simulink model "smc_diff_with_plant_new"  (R2024b)
settings: Solver=ode1  StartTime=0.0  StopTime=30  FixedStep=1e-5  RelTol=1e-3
libraries: simulink x1
settings Model: Creator=user  LastModifiedBy=user

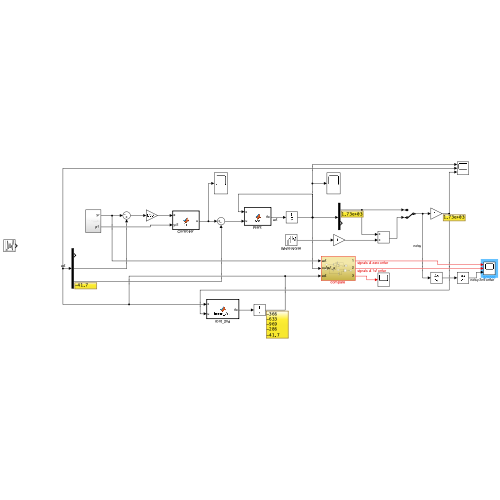
[thumbnail: Simulink's stored preview of the top-level diagram]
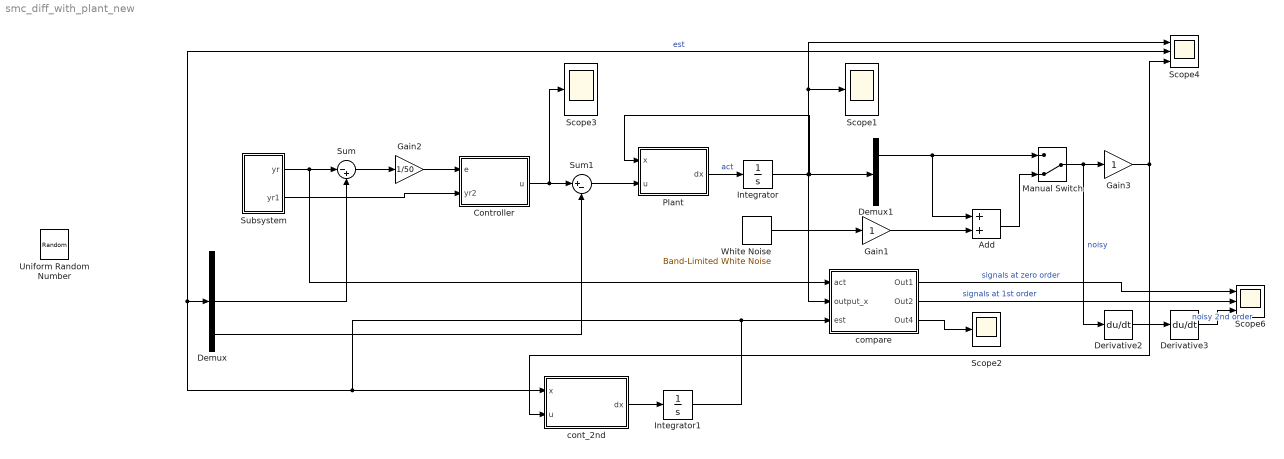
== system smc_diff_with_plant_new ==
  Add : Sum
  Controller : MATLAB Function  TreatAsAtomicUnit=on
  Demux : Demux  Outputs=[2, 2, 1]
  Demux1 : Demux  Outputs=[1, 2]
  Derivative2 : Derivative
  Derivative3 : Derivative
  Gain1 : Gain
  Gain2 : Gain  Gain=1/50
  Gain3 : Gain
  Integrator : Integrator
  Integrator1 : Integrator
  Manual Switch : ManualSwitch  CurrentSetting=0
  Plant : MATLAB Function  TreatAsAtomicUnit=on
  Scope1 : Scope
  Scope2 : Scope
  Scope3 : Scope
  Scope4 : Scope  NumInputPorts=3
  Scope6 : Scope  NumInputPorts=3
  Subsystem : Subsystem
  Sum : Sum  Inputs=|-+
  Sum1 : Sum  Inputs=|+-
  Uniform Random Number : UniformRandomNumber  Minimum=-1e-3  Maximum=1e-3  SampleTime=0.001
  White Noise : simulink/Sources/Band-Limited White Noise  Cov=1e-3*0  Ts=0.001  seed=[23341]
  compare : Subsystem
  cont_2nd : MATLAB Function  TreatAsAtomicUnit=on
  wires:
  Manual Switch/1 -> Derivative2/1, Gain3/1  "noisy"
  Gain3/1 -> cont_2nd/2(u), Scope4/3
  compare/3(Out4) -> Scope2/1
  Add/1 -> Manual Switch/2
  compare/2(Out2) -> Scope6/2  "signals at 1st order"
  Gain1/1 -> Add/2
  Derivative3/1 -> Scope6/3  "noisy 2nd order"
  Demux1/1 -> Add/1, Manual Switch/1
  White Noise/1 -> Gain1/1
  Derivative2/1 -> Derivative3/1
  Integrator/1 -> compare/2(output_x), Plant/1(x), Demux1/1, Scope1/1, Scope4/1
  Plant/1(dx) -> Integrator/1  "act"
  Sum1/1 -> Plant/2(u)
  Sum/1 -> Gain2/1
  Controller/1(u) -> Scope3/1, Sum1/1
  cont_2nd/1(dx) -> Integrator1/1
  Subsystem/2(yr1) -> Controller/2(yr2)
  Gain2/1 -> Controller/1(e)
  compare/1(Out1) -> Scope6/1  "signals at zero order"
  Demux/2 -> Sum/2
  Subsystem/1(yr) -> Sum/1, compare/1(act)
  Integrator1/1 -> Scope4/2, Demux/1, cont_2nd/1(x), compare/3(est)  "est"
  Demux/3 -> Sum1/2

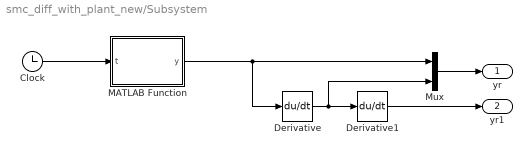
== system smc_diff_with_plant_new/Subsystem ==
  Clock : Clock
  Derivative : Derivative
  Derivative1 : Derivative
  MATLAB Function : MATLAB Function  TreatAsAtomicUnit=on
  Mux : Mux  Inputs=2
  yr : Outport
  yr1 : Outport  Port=2
  wires:
  Derivative1/1 -> yr1/1
  MATLAB Function/1(y) -> Derivative/1, Mux/1
  Derivative/1 -> Mux/2, Derivative1/1
  Mux/1 -> yr/1
  Clock/1 -> MATLAB Function/1(t)

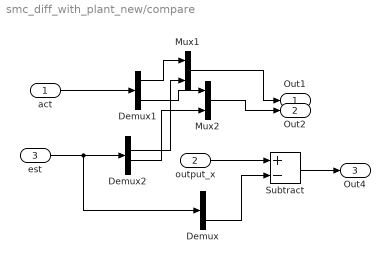
== system smc_diff_with_plant_new/compare ==
  act : Inport
  output_x : Inport  Port=2
  est : Inport  Port=3
  Demux : Demux  Outputs=[2, 3]
  Demux1 : Demux  Outputs=2
  Demux2 : Demux  Outputs=[2 1 1 1]
  Mux1 : Mux  Inputs=2
  Mux2 : Mux  Inputs=2
  Subtract : Sum  Inputs=+-
  Out1 : Outport
  Out2 : Outport  Port=2
  Out4 : Outport  Port=3
  wires:
  act/1 -> Demux1/1
  Demux1/2 -> Mux2/1
  Demux1/1 -> Mux1/1
  Mux1/1 -> Out1/1
  Demux2/2 -> Mux1/2
  est/1 -> Demux/1, Demux2/1
  Mux2/1 -> Out2/1
  Demux2/3 -> Mux2/2
  output_x/1 -> Subtract/1
  Subtract/1 -> Out4/1
  Demux/2 -> Subtract/2

== matlab function smc_diff_with_plant_new/Controller ==
  data: e input; u output; yr2 input
function u = fcn(e, yr2)
K = 20;
Iy = 0.02;
alpha = 1/Iy;
K2 = 10;
lambda = 5;
L1 = 2; L2 = 1;
s = e(2) + lambda*e(1);
ds = -L1*(abs(s)^(1/2))*sign(s) - L2*sign(s);
u = -(-yr2 + lambda*e(2) + K*sign(s) + K2*sign(ds));

== matlab function smc_diff_with_plant_new/Plant ==
  data: x input; dx output; u input
function dx = fcn(x, u)
% x = [x1; x2; f]
Iy = 0.02; % moment
beta = 0.05; % drag coeff
dx = zeros(3,1);
A = [0 1 0;
      0 0 1;
      0 0 0];
B = [0; 1/Iy; 0];
F = [0; 0; 1/Iy];
C = [1; 0; 0];

dx = A*x + B*u - F*beta*x(2);

== matlab function smc_diff_with_plant_new/Subsystem/MATLAB Function ==
  data: t input; y output
function y = fcn(t)

y = -cos(t)/(2+sin(3*t));

== matlab function smc_diff_with_plant_new/cont_2nd ==
  data: x input; u input; dx output
function dx = hosm_2nd(x, u)

%
dx = zeros(5, 1);
L = 35; % Lipschetz boundary
gamma = 1;
lambda = [1.1 3.06, 4.16 3];

z_m2 = x(1);   % z_{-2}
z_m1 = x(2);   % z_{-1}
z0   = x(3);   % z_0, estimate of u_eq
z1   = x(4);   % z_1, estimate of u_eq derivative
z2   = x(5);   % z_2, estimate of u_eq second derivative

% Extract lambda parameters:
lambda0 = lambda(1);
lambda1 = lambda(2);
lambda2 = lambda(3);
lambda3 = lambda(4);

% error
e = z_m1 - z_m2;

% Define the fractional power function:
% fpower(w, alpha) = |w|^alpha * sign(w)
fpower = @(w, alpha) (abs(w)^alpha) * sign(w);


dz_m2 = u - gamma * z_m2;

dz_m1 = -lambda3 * L^(1/4) * fpower(e, 3/4) + z0 - gamma * z_m2;
dz0   = -lambda2 * L^(2/4) * fpower(e, 2/4) + z1;
dz1   = -lambda1 * L^(3/4) * fpower(e, 1/4) + z2;
dz2   = -lambda0 * L * sign(e);

%-----------------------------------------------------------------------
% Assemble the state derivative vector:
dx = [dz_m2; dz_m1; dz0; dz1; dz2];

end
